simulink model "HemoDialysisMachine_SequenceDiagram"  (R2023a)
settings: Solver=VariableStepAuto  StartTime=0.0  StopTime=10.0  RelTol=1e-3
undefined symbols (not defined in the file): patientInfo, rising
settings Model: Creator=ppatel  LastModifiedBy=ppatel

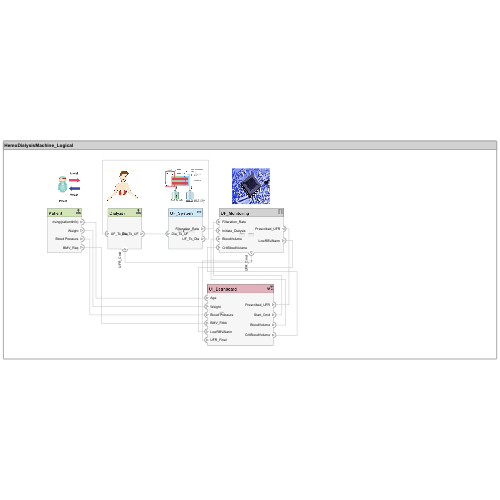
[thumbnail: Simulink's stored preview of the top-level diagram]
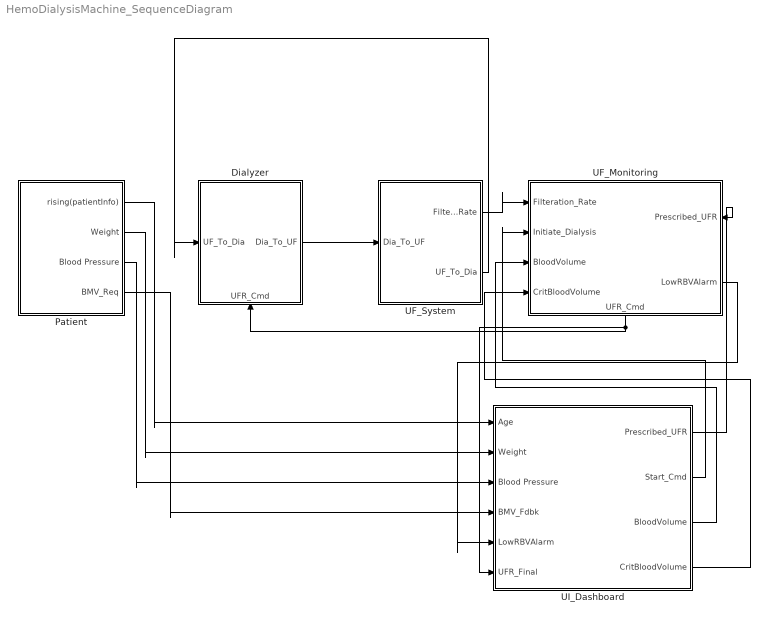
== system HemoDialysisMachine_SequenceDiagram ==
  Dialyzer : Subsystem
      settings: PortSchema="{\"entries\":[{\"content\":{\"headerSize\":26,\"margin\":15,\"minimumSpacing\":25,\"sides\":[{\"content\":{\"connectorIds\":[\"In2\"]},\"type\":\"ConnectorPlacement.EquallySpacedRectSide\",\"uuid\":\"c448f8e9-f718-4d55-8ae9-400f94c3ed78\"},{\"content\":{\"connectorIds\":[\"Out1\"],\"side\":\"RIGHT\"},\"type\":\"ConnectorPlacement.EquallySpacedRectSide\",\"uuid\":\"ddea2424-6372-4e6c-88b3-edcc675d5c44\"},{\"content\":{\"side\":\"TOP\"},\"type\":\"ConnectorPlacement.EquallySpacedRectSide\",\"uuid\":\"5d354b5e-50bd-48d5-b50b-494e2a22bc78\"},{\"content\":{\"connectorIds\":[\"In1\"],\"side\":\"BOTTOM\"},\"type\":\"ConnectorPlacement.EquallySpacedRectSide\",\"uuid\":\"60fe1de6-6664-4895-8878-6d4f8361c3a7\"}]},\"type\":\"ConnectorPlacement.EquallySpacedConnector\",\"uuid\":\"86ba679c-83d4-47d3-bf8e-52e917b1fb5f\"}],\"packageUris\":[\"http://schema.mathworks.com/mf0/Connector/R2020b\"],\"version\":\"1.0\"}"
  Patient : Subsystem
      settings: PortSchema="{\"entries\":[{\"content\":{\"headerSize\":26,\"margin\":15,\"minimumSpacing\":25,\"sides\":[{\"content\":{},\"type\":\"ConnectorPlacement.EquallySpacedRectSide\",\"uuid\":\"c448f8e9-f718-4d55-8ae9-400f94c3ed78\"},{\"content\":{\"connectorIds\":[\"Out2\",\"Out1\",\"Out3\",\"Out4\"],\"side\":\"RIGHT\"},\"type\":\"ConnectorPlacement.EquallySpacedRectSide\",\"uuid\":\"ddea2424-6372-4e6c-88b3-edcc675d5c44\"},{\"content\":{\"side\":\"TOP\"},\"type\":\"ConnectorPlacement.EquallySpacedRectSide\",\"uuid\":\"5d354b5e-50bd-48d5-b50b-494e2a22bc78\"},{\"content\":{\"side\":\"BOTTOM\"},\"type\":\"ConnectorPlacement.EquallySpacedRectSide\",\"uuid\":\"88796682-fa10-4ce9-9062-498094082345\"}]},\"type\":\"ConnectorPlacement.EquallySpacedConnector\",\"uuid\":\"86ba679c-83d4-47d3-bf8e-52e917b1fb5f\"}],\"packageUris\":[\"http://schema.mathworks.com/mf0/Connector/R2020b\"],\"version\":\"1.0\"}"
  UF_Monitoring : Subsystem
      settings: PortSchema="{\"entries\":[{\"content\":{\"headerSize\":26,\"margin\":15,\"minimumSpacing\":25,\"sides\":[{\"content\":{\"connectorIds\":[\"In1\",\"In3\",\"In4\",\"In5\"]},\"type\":\"ConnectorPlacement.EquallySpacedRectSide\",\"uuid\":\"c448f8e9-f718-4d55-8ae9-400f94c3ed78\"},{\"content\":{\"connectorIds\":[\"In2\",\"Out2\"],\"side\":\"RIGHT\"},\"type\":\"ConnectorPlacement.EquallySpacedRectSide\",\"uuid\":\"ddea2424-6372-4e6c-88b3-edcc675d5c44\"},{\"content\":{\"side\":\"TOP\"},\"type\":\"ConnectorPlacement.EquallySpacedRectSide\",\"uuid\":\"5d354b5e-50bd-48d5-b50b-494e2a22bc78\"},{\"content\":{\"connectorIds\":[\"Out1\"],\"side\":\"BOTTOM\"},\"type\":\"ConnectorPlacement.EquallySpacedRectSide\",\"uuid\":\"50ece032-5537-489c-8a4a-ab4621a78d52\"}]},\"type\":\"ConnectorPlacement.EquallySpacedConnector\",\"uuid\":\"86ba679c-83d4-47d3-bf8e-52e917b1fb5f\"}],\"packageUris\":[\"http://schema.mathworks.com/mf0/Connector/R2020b\"],\"version\":\"1.0\"}"
  UF_System : Subsystem
      settings: PortSchema="{\"entries\":[{\"content\":{\"headerSize\":26,\"margin\":15,\"minimumSpacing\":25,\"sides\":[{\"content\":{\"connectorIds\":[\"In1\"]},\"type\":\"ConnectorPlacement.EquallySpacedRectSide\",\"uuid\":\"c448f8e9-f718-4d55-8ae9-400f94c3ed78\"},{\"content\":{\"connectorIds\":[\"Out1\",\"Out2\"],\"side\":\"RIGHT\"},\"type\":\"ConnectorPlacement.EquallySpacedRectSide\",\"uuid\":\"ddea2424-6372-4e6c-88b3-edcc675d5c44\"},{\"content\":{\"side\":\"TOP\"},\"type\":\"ConnectorPlacement.EquallySpacedRectSide\",\"uuid\":\"5d354b5e-50bd-48d5-b50b-494e2a22bc78\"}]},\"type\":\"ConnectorPlacement.EquallySpacedConnector\",\"uuid\":\"86ba679c-83d4-47d3-bf8e-52e917b1fb5f\"}],\"packageUris\":[\"http://schema.mathworks.com/mf0/Connector/R2020b\"],\"version\":\"1.0\"}"
  UI_Dashboard : Subsystem
      settings: PortSchema="{\"entries\":[{\"content\":{\"headerSize\":26,\"margin\":15,\"minimumSpacing\":25,\"sides\":[{\"content\":{\"connectorIds\":[\"In1\",\"In2\",\"In3\",\"In4\",\"In5\",\"In6\"]},\"type\":\"ConnectorPlacement.EquallySpacedRectSide\",\"uuid\":\"c448f8e9-f718-4d55-8ae9-400f94c3ed78\"},{\"content\":{\"connectorIds\":[\"Out1\",\"Out2\",\"Out3\",\"Out4\"],\"side\":\"RIGHT\"},\"type\":\"ConnectorPlacement.EquallySpacedRectSide\",\"uuid\":\"ddea2424-6372-4e6c-88b3-edcc675d5c44\"},{\"content\":{\"side\":\"TOP\"},\"type\":\"ConnectorPlacement.EquallySpacedRectSide\",\"uuid\":\"5d354b5e-50bd-48d5-b50b-494e2a22bc78\"}]},\"type\":\"ConnectorPlacement.EquallySpacedConnector\",\"uuid\":\"86ba679c-83d4-47d3-bf8e-52e917b1fb5f\"}],\"packageUris\":[\"http://schema.mathworks.com/mf0/Connector/R2020b\"],\"version\":\"1.0\"}"
  wires:
  Dialyzer/1(Dia_To_UF) -> UF_System/1(Dia_To_UF)
  UF_Monitoring/1(UFR_Cmd) -> UI_Dashboard/6(UFR_Final), Dialyzer/1(UFR_Cmd)
  Patient/1(Weight) -> UI_Dashboard/2(Weight)
  Patient/2(rising(patientInfo)) -> UI_Dashboard/1(Age)
  Patient/3(Blood Pressure) -> UI_Dashboard/3(Blood Pressure)
  UI_Dashboard/1(Prescribed_UFR) -> UF_Monitoring/2(Prescribed_UFR)
  UF_System/1(Filteration_Rate) -> UF_Monitoring/1(Filteration_Rate)
  UI_Dashboard/2(Start_Cmd) -> UF_Monitoring/3(Initiate_Dialysis)
  UF_System/2(UF_To_Dia) -> Dialyzer/2(UF_To_Dia)
  Patient/4(BMV_Req) -> UI_Dashboard/4(BMV_Fdbk)
  UI_Dashboard/3(BloodVolume) -> UF_Monitoring/4(BloodVolume)
  UI_Dashboard/4(CritBloodVolume) -> UF_Monitoring/5(CritBloodVolume)
  UF_Monitoring/2(LowRBVAlarm) -> UI_Dashboard/5(LowRBVAlarm)

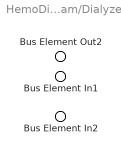
== system HemoDialysisMachine_SequenceDiagram/Dialyzer ==
  Bus Element In1 : Inport  PortName=UFR_Cmd
  Bus Element In2 : Inport  Port=2  PortName=UF_To_Dia
  Bus Element Out2 : Outport  PortName=Dia_To_UF

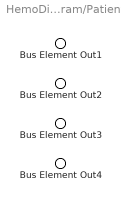
== system HemoDialysisMachine_SequenceDiagram/Patient ==
  Bus Element Out1 : Outport  PortName=Weight
  Bus Element Out2 : Outport  Port=2  PortName=rising(patientInfo)
  Bus Element Out3 : Outport  Port=3  PortName=Blood Pressure
  Bus Element Out4 : Outport  Port=4  PortName=BMV_Req

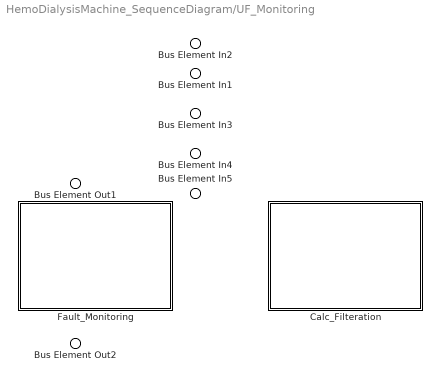
== system HemoDialysisMachine_SequenceDiagram/UF_Monitoring ==
  Bus Element In1 : Inport  PortName=Filteration_Rate
  Bus Element In2 : Inport  Port=2  PortName=Prescribed_UFR
  Bus Element In3 : Inport  Port=3  PortName=Initiate_Dialysis
  Bus Element In4 : Inport  Port=4  PortName=BloodVolume
  Bus Element In5 : Inport  Port=5  PortName=CritBloodVolume
  Calc_Filteration : Subsystem
      settings: PortSchema="{\"entries\":[{\"content\":{\"headerSize\":26,\"margin\":15,\"minimumSpacing\":25,\"sides\":[{\"content\":{},\"type\":\"ConnectorPlacement.EquallySpacedRectSide\",\"uuid\":\"c448f8e9-f718-4d55-8ae9-400f94c3ed78\"},{\"content\":{\"side\":\"RIGHT\"},\"type\":\"ConnectorPlacement.EquallySpacedRectSide\",\"uuid\":\"ddea2424-6372-4e6c-88b3-edcc675d5c44\"},{\"content\":{\"side\":\"TOP\"},\"type\":\"ConnectorPlacement.EquallySpacedRectSide\",\"uuid\":\"5d354b5e-50bd-48d5-b50b-494e2a22bc78\"}]},\"type\":\"ConnectorPlacement.EquallySpacedConnector\",\"uuid\":\"86ba679c-83d4-47d3-bf8e-52e917b1fb5f\"}],\"packageUris\":[\"http://schema.mathworks.com/mf0/Connector/R2020b\"],\"version\":\"1.0\"}"
  Fault_Monitoring : Subsystem
      settings: PortSchema="{\"entries\":[{\"content\":{\"headerSize\":26,\"margin\":15,\"minimumSpacing\":25,\"sides\":[{\"content\":{},\"type\":\"ConnectorPlacement.EquallySpacedRectSide\",\"uuid\":\"a687e012-4840-413d-ae7b-c05f2b55ca05\"},{\"content\":{\"side\":\"RIGHT\"},\"type\":\"ConnectorPlacement.EquallySpacedRectSide\",\"uuid\":\"6a695777-1bf4-4cf6-ae1b-4fd6cbf201ea\"},{\"content\":{\"side\":\"TOP\"},\"type\":\"ConnectorPlacement.EquallySpacedRectSide\",\"uuid\":\"4e0efd68-4a3d-4565-a916-e6cda3743f29\"}]},\"type\":\"ConnectorPlacement.EquallySpacedConnector\",\"uuid\":\"de7bea47-d1da-4071-a467-1cf916758324\"}],\"packageUris\":[\"http://schema.mathworks.com/mf0/Connector/R2020b\"],\"version\":\"1.0\"}"
  Bus Element Out1 : Outport  PortName=UFR_Cmd
  Bus Element Out2 : Outport  Port=2  PortName=LowRBVAlarm

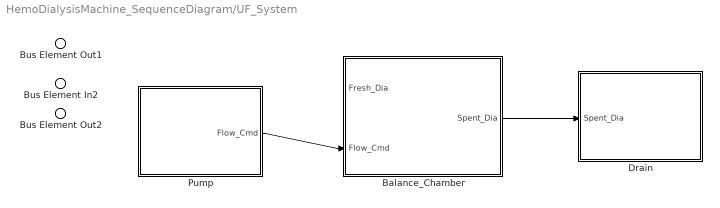
== system HemoDialysisMachine_SequenceDiagram/UF_System ==
  Bus Element In2 : Inport  PortName=Dia_To_UF
  Balance_Chamber : Subsystem
      settings: PortSchema="{\"entries\":[{\"content\":{\"headerSize\":26,\"margin\":15,\"minimumSpacing\":25,\"sides\":[{\"content\":{\"connectorIds\":[\"In1\",\"In2\"]},\"type\":\"ConnectorPlacement.EquallySpacedRectSide\",\"uuid\":\"c448f8e9-f718-4d55-8ae9-400f94c3ed78\"},{\"content\":{\"connectorIds\":[\"Out1\"],\"side\":\"RIGHT\"},\"type\":\"ConnectorPlacement.EquallySpacedRectSide\",\"uuid\":\"ddea2424-6372-4e6c-88b3-edcc675d5c44\"},{\"content\":{\"side\":\"TOP\"},\"type\":\"ConnectorPlacement.EquallySpacedRectSide\",\"uuid\":\"5d354b5e-50bd-48d5-b50b-494e2a22bc78\"}]},\"type\":\"ConnectorPlacement.EquallySpacedConnector\",\"uuid\":\"86ba679c-83d4-47d3-bf8e-52e917b1fb5f\"}],\"packageUris\":[\"http://schema.mathworks.com/mf0/Connector/R2020b\"],\"version\":\"1.0\"}"
  Drain : Subsystem
      settings: PortSchema="{\"entries\":[{\"content\":{\"headerSize\":26,\"margin\":15,\"minimumSpacing\":25,\"sides\":[{\"content\":{\"connectorIds\":[\"In1\"]},\"type\":\"ConnectorPlacement.EquallySpacedRectSide\",\"uuid\":\"c448f8e9-f718-4d55-8ae9-400f94c3ed78\"},{\"content\":{\"side\":\"RIGHT\"},\"type\":\"ConnectorPlacement.EquallySpacedRectSide\",\"uuid\":\"ddea2424-6372-4e6c-88b3-edcc675d5c44\"},{\"content\":{\"side\":\"TOP\"},\"type\":\"ConnectorPlacement.EquallySpacedRectSide\",\"uuid\":\"5d354b5e-50bd-48d5-b50b-494e2a22bc78\"}]},\"type\":\"ConnectorPlacement.EquallySpacedConnector\",\"uuid\":\"86ba679c-83d4-47d3-bf8e-52e917b1fb5f\"}],\"packageUris\":[\"http://schema.mathworks.com/mf0/Connector/R2020b\"],\"version\":\"1.0\"}"
  Pump : Subsystem
      settings: PortSchema="{\"entries\":[{\"content\":{\"headerSize\":26,\"margin\":15,\"minimumSpacing\":25,\"sides\":[{\"content\":{},\"type\":\"ConnectorPlacement.EquallySpacedRectSide\",\"uuid\":\"c448f8e9-f718-4d55-8ae9-400f94c3ed78\"},{\"content\":{\"connectorIds\":[\"Out1\"],\"side\":\"RIGHT\"},\"type\":\"ConnectorPlacement.EquallySpacedRectSide\",\"uuid\":\"ddea2424-6372-4e6c-88b3-edcc675d5c44\"},{\"content\":{\"side\":\"TOP\"},\"type\":\"ConnectorPlacement.EquallySpacedRectSide\",\"uuid\":\"5d354b5e-50bd-48d5-b50b-494e2a22bc78\"}]},\"type\":\"ConnectorPlacement.EquallySpacedConnector\",\"uuid\":\"86ba679c-83d4-47d3-bf8e-52e917b1fb5f\"}],\"packageUris\":[\"http://schema.mathworks.com/mf0/Connector/R2020b\"],\"version\":\"1.0\"}"
  Bus Element Out1 : Outport  PortName=Filteration_Rate
  Bus Element Out2 : Outport  Port=2  PortName=UF_To_Dia
  wires:
  Pump/1(Flow_Cmd) -> Balance_Chamber/2(Flow_Cmd)
  Balance_Chamber/1(Spent_Dia) -> Drain/1(Spent_Dia)
  ? -> Balance_Chamber/1(Fresh_Dia)

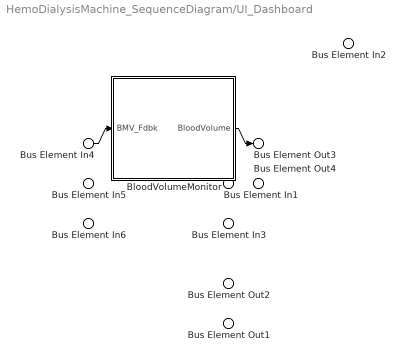
== system HemoDialysisMachine_SequenceDiagram/UI_Dashboard ==
  Bus Element In2 : Inport  PortName=Age
  Bus Element In1 : Inport  Port=2  PortName=Weight
  Bus Element In3 : Inport  Port=3  PortName=Blood Pressure
  Bus Element In4 : Inport  Port=4  PortName=BMV_Fdbk
  Bus Element In5 : Inport  Port=5  PortName=LowRBVAlarm
  Bus Element In6 : Inport  Port=6  PortName=UFR_Final
  BloodVolumeMonitor : Subsystem
      settings: PortSchema="{\"entries\":[{\"content\":{\"headerSize\":26,\"margin\":15,\"minimumSpacing\":25,\"sides\":[{\"content\":{\"connectorIds\":[\"In1\"]},\"type\":\"ConnectorPlacement.EquallySpacedRectSide\",\"uuid\":\"26d21b59-92b1-4efd-afff-4bac4af91e92\"},{\"content\":{\"connectorIds\":[\"Out1\"],\"side\":\"RIGHT\"},\"type\":\"ConnectorPlacement.EquallySpacedRectSide\",\"uuid\":\"874338f8-5b85-4580-9930-3f474badb449\"},{\"content\":{\"side\":\"TOP\"},\"type\":\"ConnectorPlacement.EquallySpacedRectSide\",\"uuid\":\"3c09baea-9cf4-48aa-ae56-dcfb9b28f106\"}]},\"type\":\"ConnectorPlacement.EquallySpacedConnector\",\"uuid\":\"2527176d-f071-40a3-bd13-d8fac6b76ca1\"}],\"packageUris\":[\"http://schema.mathworks.com/mf0/Connector/R2020b\"],\"version\":\"1.0\"}"
  Bus Element Out2 : Outport  PortName=Prescribed_UFR
  Bus Element Out1 : Outport  Port=2  PortName=Start_Cmd
  Bus Element Out3 : Outport  Port=3  PortName=BloodVolume
  Bus Element Out4 : Outport  Port=4  PortName=CritBloodVolume
  wires:
  Bus Element In4/1 -> BloodVolumeMonitor/1(BMV_Fdbk)
  BloodVolumeMonitor/1(BloodVolume) -> Bus Element Out3/1

== system HemoDialysisMachine_SequenceDiagram/UF_Monitoring/Calc_Filteration ==

== system HemoDialysisMachine_SequenceDiagram/UF_Monitoring/Fault_Monitoring ==

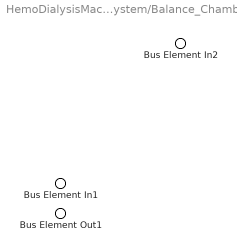
== system HemoDialysisMachine_SequenceDiagram/UF_System/Balance_Chamber ==
  Bus Element In2 : Inport  PortName=Fresh_Dia
  Bus Element In1 : Inport  Port=2  PortName=Flow_Cmd
  Bus Element Out1 : Outport  PortName=Spent_Dia

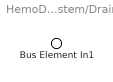
== system HemoDialysisMachine_SequenceDiagram/UF_System/Drain ==
  Bus Element In1 : Inport  PortName=Spent_Dia

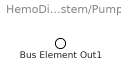
== system HemoDialysisMachine_SequenceDiagram/UF_System/Pump ==
  Bus Element Out1 : Outport  PortName=Flow_Cmd

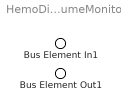
== system HemoDialysisMachine_SequenceDiagram/UI_Dashboard/BloodVolumeMonitor ==
  Bus Element In1 : Inport  PortName=BMV_Fdbk
  Bus Element Out1 : Outport  PortName=BloodVolume
